simulink model "c_d"  (R2015a)
settings: Solver=ode45  StartTime=0.0  StopTime=10.0  RelTol=1e-3
settings Model: Creator=luis  LastModifiedBy=Dany
settings DataIOCC: SignalLoggingSaveFormat=ModelDataLogs
settings OptimizationCC: ExpressionDepthLimit=2147483647
settings DebuggingCC: UnderspecifiedInitializationDetection=Classic  MergeDetectMultiDrivingBlocksExec=none  SolverPrmCheckMsg=warning  FcnCallInpInsideContextMsg=EnableAllAsWarning  StateNameClashWarn=warning

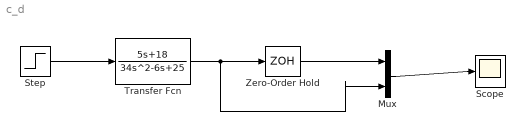
== system c_d ==
  Mux : Mux  Inputs=2
  Scope : Scope
      settings: TickLabels=on
  Step : Step  SampleTime=0
  Transfer Fcn : TransferFcn  Numerator=[5 18]  Denominator=[34 -6 25]
  Zero-Order Hold : ZeroOrderHold  SampleTime=0.08
  wires:
  Step/1 -> Transfer Fcn/1
  Transfer Fcn/1 -> Zero-Order Hold/1, Mux/2
  Zero-Order Hold/1 -> Mux/1
  Mux/1 -> Scope/1
